simulink model "ZRM"  (R2021a)
settings: Solver=ode8  StartTime=0.0  StopTime=10.0  RelTol=1e-3
model workspace (MAT data in the model file):
  A = Simulink.Parameter
  A.Value = [0  1; 0  0]
  A.DataType = 'auto'
  A.Complexity = 'real'
  A.Dimensions = [2 2]
  B = Simulink.Parameter
  B.Value = 0.3
  B.DataType = 'auto'
  B.Complexity = 'real'
  B.Dimensions = [1 1]
  C = Simulink.Parameter
  C.Value = [1 0]
  C.DataType = 'auto'
  C.Complexity = 'real'
  C.Dimensions = [1 2]
  x0 = Simulink.Parameter
  x0.DataType = 'auto'
  x0.Complexity = 'real'
  x0.Dimensions = [0 0]
settings Model: ParameterArgumentNames=B  Creator=Hoorsana  LastModifiedBy=Hoorsana

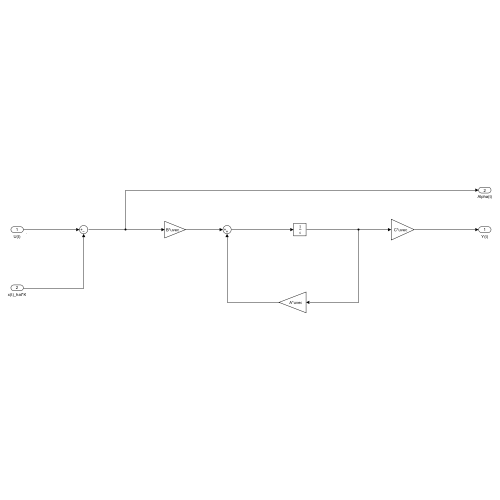
[thumbnail: Simulink's stored preview of the top-level diagram]
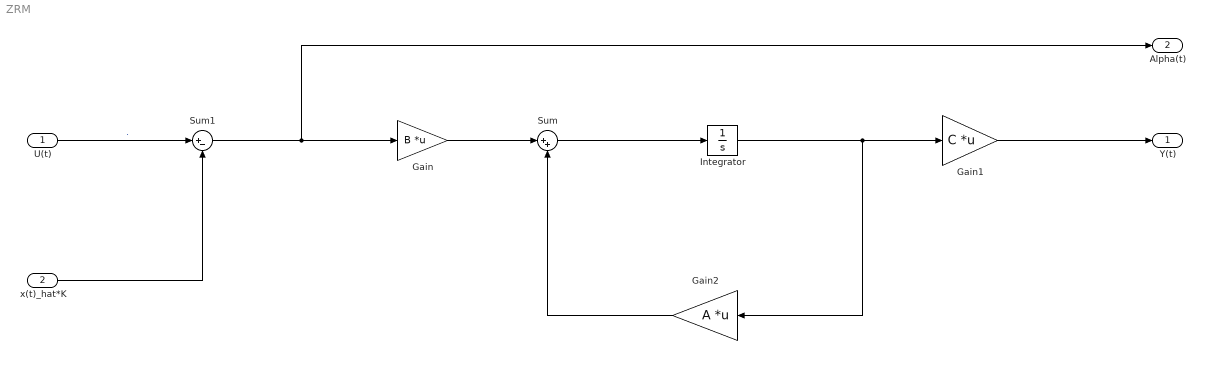
== system ZRM ==
  U(t) : Inport
  x(t)_hat*K : Inport  Port=2
  Gain : Gain  Gain=B  Multiplication=Matrix(K*u) (u vector)
  Gain1 : Gain  Gain=C  Multiplication=Matrix(K*u) (u vector)
  Gain2 : Gain  Gain=A  Multiplication=Matrix(K*u) (u vector)
  Integrator : Integrator  InitialCondition=0.3
  Sum : Sum  Inputs=|++
  Sum1 : Sum  Inputs=|+-
  Y(t) : Outport  VectorParamsAs1DForOutWhenUnconnected=off
  Alpha(t) : Outport  Port=2  VectorParamsAs1DForOutWhenUnconnected=off
  wires:
  Gain1/1 -> Y(t)/1
  Integrator/1 -> Gain2/1, Gain1/1
  x(t)_hat*K/1 -> Sum1/2
  Gain/1 -> Sum/1
  U(t)/1 -> Sum1/1  "."
  Sum1/1 -> Alpha(t)/1, Gain/1
  Sum/1 -> Integrator/1
  Gain2/1 -> Sum/2
